simulink model "Modelll_1"  (Simulink 9.2)
settings: Solver=ode23  StartTime=0.0  StopTime=10.0  RelTol=1e-3
values from neighbouring files (symbols this model uses):
  a = 0.5    [aufgabe_2.m]
  b = 0.75    [aufgabe_2.m]
  w = 2    [Ex_3.m]    (also in aufgabe_2.m)
libraries: simulink x1
settings Model: Creator=gyant  LastModifiedBy=gyant
settings DataIOCC: LimitDataPoints=off  SaveFormat=Dataset  SignalLoggingSaveFormat=Dataset
settings OptimizationCC: LifeSpan=auto
settings DebuggingCC: UnderspecifiedInitializationDetection=Simplified  MergeDetectMultiDrivingBlocksExec=error  FcnCallInpInsideContextMsg=error  StateNameClashWarn=none  SFUnexpectedBacktrackingDiag=error  SFNoUnconditionalDefaultTransitionDiag=error  SFExecutionAtInitializationDiag=warning
settings HardwareCC: ProdBitPerPointer=64  ProdBitPerSizeT=64  ProdBitPerPtrDiffT=64  ProdLargestAtomicFloat=Float  ProdIntDivRoundTo=Zero  ProdEndianess=LittleEndian  ProdWordSize=64  ProdHWDeviceType=Intel->x86-64 (Windows64)
settings ModelReferenceCC: PropagateSignalLabelsOutOfModel=on
settings SFSimCC: SimUseLocalCustomCode=on
settings RTWCC: RTWUseLocalCustomCode=on
settings CodeAppCC: StateflowObjectComments=off
settings GRTTargetCC: TargetLangStandard=C99 (ISO)  GeneratePreprocessorConditionals=Use local settings  CombineOutputUpdateFcns=on  GRTInterface=off
settings ConfigComp: CovMetricSettings=dwe  CovHtmlReporting=off  CovSaveCumulativeToWorkspaceVar=off  CovSaveSingleToWorkspaceVar=off  CovExternalEMLEnable=on

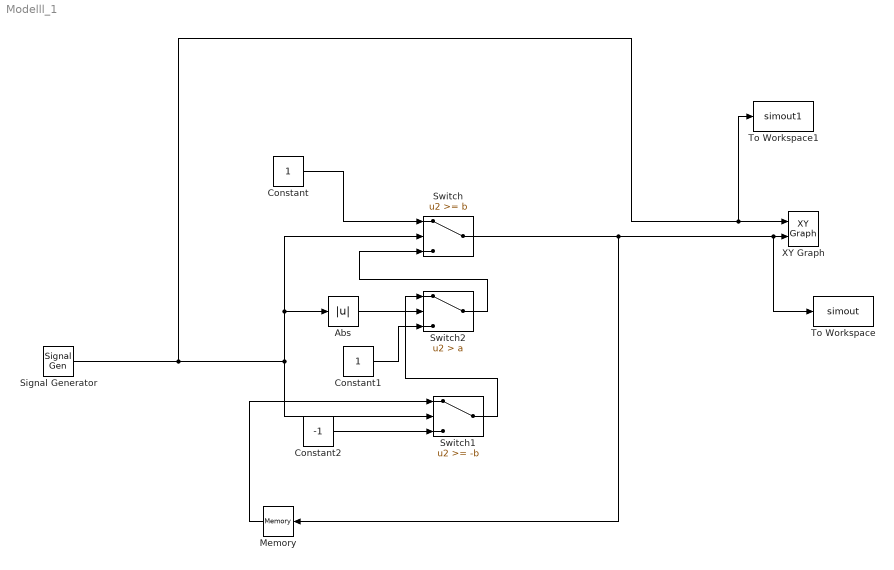
== system Modelll_1 ==
  Abs : Abs
  Constant : Constant
  Constant1 : Constant
  Constant2 : Constant  Value=-1
  Memory : Memory
  Signal Generator : SignalGenerator  Frequency=w  Units=rad/sec
  Switch : Switch  Threshold=b
  Switch1 : Switch  Threshold=-b
  Switch2 : Switch  Criteria=u2 > Threshold  Threshold=a
  To Workspace : ToWorkspace  VariableName=simout  SaveFormat=Structure With Time  SampleTime=-1
  To Workspace1 : ToWorkspace  VariableName=simout1  SaveFormat=Structure  SampleTime=-1
  XY Graph : simulink/Sinks/XY Graph  xmin=-2  xmax=1  ymin=-1  ymax=1  st=-1
  wires:
  Signal Generator/1 -> Switch/2, Abs/1, Switch1/2, To Workspace1/1, XY Graph/1
  Constant/1 -> Switch/1
  Switch/1 -> To Workspace/1, XY Graph/2, Memory/1
  Switch2/1 -> Switch/3
  Abs/1 -> Switch2/2
  Constant1/1 -> Switch2/3
  Constant2/1 -> Switch1/3
  Memory/1 -> Switch1/1
  Switch1/1 -> Switch2/1
